simulink model "gain_test_ElementWise"  (Simulink 7.2)
settings: Solver=ode3  StartTime=0.0  StopTime=10.0  FixedStep=0.1  RelTol=1e-3
settings Model: Creator=arnaud  LastModifiedBy=arnaud
settings DataIOCC: SaveFormat=Structure
settings DebuggingCC: UnnecessaryDatatypeConvMsg=warning  VectorMatrixConversionMsg=warning

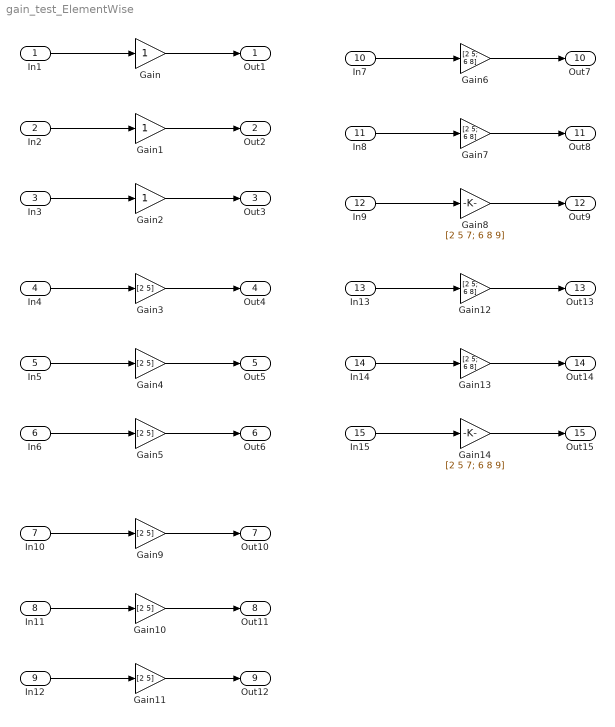
== system gain_test_ElementWise ==
  In1 : Inport  DataType=double  OutDataType=sfix(16)  OutScaling=2^0  OutDataTypeStr=double
  In2 : Inport  Port=2  DataType=int8  OutDataType=sfix(16)  OutScaling=2^0  OutDataTypeStr=int8
  In3 : Inport  Port=3  DataType=boolean  OutDataType=sfix(16)  OutScaling=2^0  OutDataTypeStr=boolean
  In4 : Inport  Port=4  PortDimensions=1  DataType=double  OutDataType=sfix(16)  OutScaling=2^0  OutDataTypeStr=double
  In5 : Inport  Port=5  PortDimensions=1  DataType=int8  OutDataType=sfix(16)  OutScaling=2^0  OutDataTypeStr=int8
  In6 : Inport  Port=6  PortDimensions=1  DataType=boolean  OutDataType=sfix(16)  OutScaling=2^0  OutDataTypeStr=boolean
  In10 : Inport  Port=7  PortDimensions=2  DataType=double  OutDataType=sfix(16)  OutScaling=2^0  OutDataTypeStr=double
  In11 : Inport  Port=8  PortDimensions=2  DataType=int8  OutDataType=sfix(16)  OutScaling=2^0  OutDataTypeStr=int8
  In12 : Inport  Port=9  PortDimensions=2  DataType=boolean  OutDataType=sfix(16)  OutScaling=2^0  OutDataTypeStr=boolean
  In7 : Inport  Port=10  PortDimensions=1  DataType=double  OutDataType=sfix(16)  OutScaling=2^0  OutDataTypeStr=double
  In8 : Inport  Port=11  PortDimensions=1  DataType=int8  OutDataType=sfix(16)  OutScaling=2^0  OutDataTypeStr=int8
  In9 : Inport  Port=12  PortDimensions=1  DataType=boolean  OutDataType=sfix(16)  OutScaling=2^0  OutDataTypeStr=boolean
  In13 : Inport  Port=13  PortDimensions=[2 2]  DataType=double  OutDataType=sfix(16)  OutScaling=2^0  OutDataTypeStr=double
  In14 : Inport  Port=14  PortDimensions=[2 2]  DataType=int8  OutDataType=sfix(16)  OutScaling=2^0  OutDataTypeStr=int8
  In15 : Inport  Port=15  PortDimensions=[2 3]  DataType=boolean  OutDataType=sfix(16)  OutScaling=2^0  OutDataTypeStr=boolean
  Gain : Gain  ParameterDataType=sfix(16)  ParameterScaling=2^0  OutDataType=sfix(16)  OutScaling=2^0
  Gain1 : Gain  ParameterDataType=sfix(16)  ParameterScaling=2^0  OutDataType=sfix(16)  OutScaling=2^0
  Gain{3..5,9..11} (6 alike) : Gain  Gain=[2 5]  ParameterDataType=sfix(16)  ParameterScaling=2^0  OutDataType=sfix(16)  OutScaling=2^0
  Gain{6..7,12..13} (4 alike) : Gain  Gain=[2 5; 6 8]  ParameterDataType=sfix(16)  ParameterScaling=2^0  OutDataType=sfix(16)  OutScaling=2^0
  Gain14 : Gain  Gain=[2 5 7; 6 8 9]  ParameterDataType=sfix(16)  ParameterScaling=2^0  OutDataType=sfix(16)  OutScaling=2^0
  Gain2 : Gain  ParameterDataType=sfix(16)  ParameterScaling=2^0  OutDataType=sfix(16)  OutScaling=2^0
  Gain8 : Gain  Gain=[2 5 7; 6 8 9]  ParameterDataType=sfix(16)  ParameterScaling=2^0  OutDataType=sfix(16)  OutScaling=2^0
  Out1 : Outport  OutDataType=sfix(16)  OutScaling=2^0
  Out2 : Outport  Port=2  OutDataType=sfix(16)  OutScaling=2^0
  Out3 : Outport  Port=3  OutDataType=sfix(16)  OutScaling=2^0
  Out4 : Outport  Port=4  OutDataType=sfix(16)  OutScaling=2^0
  Out5 : Outport  Port=5  OutDataType=sfix(16)  OutScaling=2^0
  Out6 : Outport  Port=6  OutDataType=sfix(16)  OutScaling=2^0
  Out10 : Outport  Port=7  OutDataType=sfix(16)  OutScaling=2^0
  Out11 : Outport  Port=8  OutDataType=sfix(16)  OutScaling=2^0
  Out12 : Outport  Port=9  OutDataType=sfix(16)  OutScaling=2^0
  Out7 : Outport  Port=10  OutDataType=sfix(16)  OutScaling=2^0
  Out8 : Outport  Port=11  OutDataType=sfix(16)  OutScaling=2^0
  Out9 : Outport  Port=12  OutDataType=sfix(16)  OutScaling=2^0
  Out13 : Outport  Port=13  OutDataType=sfix(16)  OutScaling=2^0
  Out14 : Outport  Port=14  OutDataType=sfix(16)  OutScaling=2^0
  Out15 : Outport  Port=15  OutDataType=sfix(16)  OutScaling=2^0
  wires:
  In1/1 -> Gain/1
  Gain/1 -> Out1/1
  In2/1 -> Gain1/1
  Gain1/1 -> Out2/1
  In3/1 -> Gain2/1
  Gain2/1 -> Out3/1
  In4/1 -> Gain3/1
  Gain3/1 -> Out4/1
  In5/1 -> Gain4/1
  Gain4/1 -> Out5/1
  In6/1 -> Gain5/1
  Gain5/1 -> Out6/1
  In10/1 -> Gain9/1
  Gain9/1 -> Out10/1
  In11/1 -> Gain10/1
  Gain10/1 -> Out11/1
  In12/1 -> Gain11/1
  Gain11/1 -> Out12/1
  In7/1 -> Gain6/1
  Gain6/1 -> Out7/1
  In8/1 -> Gain7/1
  Gain7/1 -> Out8/1
  In9/1 -> Gain8/1
  Gain8/1 -> Out9/1
  In13/1 -> Gain12/1
  Gain12/1 -> Out13/1
  In14/1 -> Gain13/1
  Gain13/1 -> Out14/1
  In15/1 -> Gain14/1
  Gain14/1 -> Out15/1
